simulink model "power_diode"  (Simulink 6.0)
settings: Solver=ode23tb  SolverMode=SingleTasking  StartTime=0.0  StopTime=0.06  FixedStep=100e-6  RelTol=1e-3  AbsTol=1e-2
libraries: powerlib x7
settings Model: Creator=patrice  LastModifiedBy=batserve  ExtModeTrigMode=oneshot  ExtModeArmWhenConnect=off  ExtModeAutoUpdateStatusClock=off
settings DataIOCC: LimitDataPoints=off  SaveOutput=off  SaveTime=off  TimeSaveName=t  SignalLoggingName=sigsOut
settings OptimizationCC: BlockReduction=off  BooleanDataType=off
settings DebuggingCC: SolverPrmCheckMsg=none
settings HardwareCC: TargetUnknown=on
settings RTWCC: TemplateMakefile=grt_unix.tmf

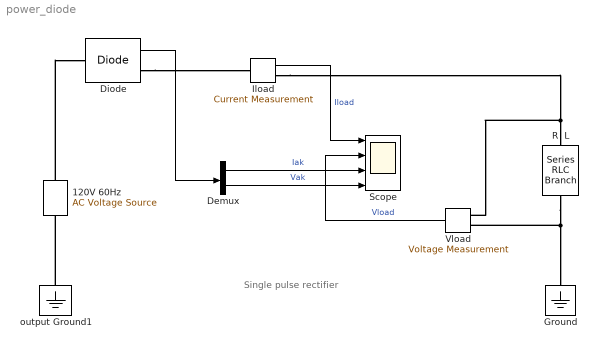
== system power_diode ==
  note: Single pulse rectifier
  120V 60Hz : powerlib/Electrical Sources/AC Voltage Source  Description=source block  Orientation=up  Amplitude=120  Phase=0  Frequency=60  SampleTime=0  Measurements=None
      settings: AttributesFormatString=\n
  Demux : Demux  Outputs=2
  Diode : powerlib/Power Electronics/Diode  Ron=0.001  Lon=1e-6  Vf=0.8  IC=0  Rs=20  Cs=4e-6  Measurements=on
  Ground : powerlib/Elements/Ground  Orientation=down  PhysicalDomain=powersysdomain  SubClassName=unknown  PortType=p1  LConnTagsString=a
  Iload : powerlib/Measurements/Current Measurement  Tag=PoWeRsYsTeMmEaSuReMeNt  PhasorSimulation=off  OutputType=Magnitude  PSBequivalent=0
  R  L : powerlib/Elements/Series RLC Branch  Orientation=down  PhysicalDomain=powersysdomain  SubClassName=unknown  PortType=p1  LConnTagsString=__new0  RConnTagsString=__new0  Resistance=1  Inductance=1e-03  Capacitance=inf  Measurements=None
  Scope : Scope  NumInputPorts=4
      settings: TimeRange=0.06  YMin=-200~-200~0~-200  YMax=200~200~200~200  DataFormat=Array
  Vload : powerlib/Measurements/Voltage Measurement  Tag=PoWeRsYsTeMmEaSuReMeNt  Orientation=left  PhasorSimulation=off  OutputType=Magnitude  PSBequivalent=0
  output Ground1 : powerlib/Elements/Ground  Orientation=down  PhysicalDomain=powersysdomain  SubClassName=unknown  PortType=p1  LConnTagsString=a
  wires:
  Demux/1 -> Scope/3  "Iak"
  Demux/2 -> Scope/4  "Vak"
  Diode/1 -> Demux/1
  Iload/1 -> Scope/1  "Iload"
  Vload/1 -> Scope/2  "Vload"
  connections:
  Iload/RConn1 -- R  L/LConn1 -- Vload/LConn1
  R  L/RConn1 -- Ground/LConn1 -- Vload/LConn2
  Diode/RConn1 -- Iload/LConn1
  output Ground1/LConn1 -- 120V 60Hz/LConn1
  120V 60Hz/RConn1 -- Diode/LConn1
